simulink model "PID_controller"  (R2020a)
settings: Solver=VariableStepAuto  StartTime=0.0  StopTime=20  MaxStep=1e-3  RelTol=1e-3  EnableMultiTasking=on
settings Model: SILPILModeSetting=veronly  ExtModeTrigDuration=2  Creator=Administrator  LastModifiedBy=Administrator
settings OptimizationCC: BlockReduction=off  EnhancedBackFolding=on  PassReuseOutputArgsAs=Individual arguments  ZeroExternalMemoryAtStartup=off  ZeroInternalMemoryAtStartup=off  MaxStackSize=64  OptimizeBlockOrder=speed  DifferentSizesBufferReuse=on  OptimizationCustomize=off  EfficientTunableParamExpr=on
settings DebuggingCC: ParameterTunabilityLossMsg=error
settings HardwareCC: ProdBitPerInt=16  ProdBitPerPointer=16  ProdBitPerSizeT=16  ProdBitPerPtrDiffT=16  ProdLargestAtomicFloat=None  ProdWordSize=8  ProdHWDeviceType=Atmel->AVR
settings SFSimCC: MATLABDynamicMemAlloc=off
settings RTWCC: SystemTargetFile=ert.tlc  HardwareBoard=Arduino Uno  TLCOptions=-aInlineSetEventsForThisBaseRateFcn=TLC_FALSE -aSuppressMultiTaskScheduler=TLC_FALSE -aRateBasedStepFcn=1  TemplateMakefile=ert_default_tmf  Toolchain=Arduino AVR  BuildConfiguration=Faster Runs
settings CodeAppCC: ForceParamTrailComments=on  IgnoreCustomStorageClasses=off  OperatorAnnotations=on  SimulinkDataObjDesc=on  SFDataObjDesc=on  InsertBlockDesc=on
settings ERTTargetCC: SupportContinuousTime=on  SupportVariableSizeSignals=on  ExtModeStaticAllocSize=250

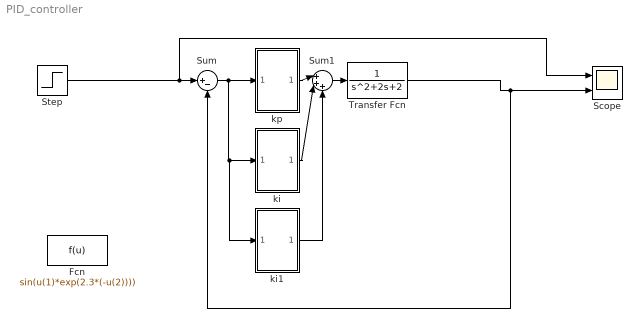
== system PID_controller ==
  Fcn : Fcn  Expr=sin(u(1)*exp(2.3*(-u(2))))
  Scope : Scope  NumInputPorts=2
  Step : Step  SampleTime=1
  Sum : Sum  Inputs=|+-
  Sum1 : Sum  Inputs=|+++
  Transfer Fcn : TransferFcn  Denominator=[1 2 2]
  ki : Subsystem
  ki1 : Subsystem
  kp : Subsystem
  wires:
  Step/1 -> Scope/1, Sum/1
  Transfer Fcn/1 -> Sum/2, Scope/2
  Sum/1 -> ki1/1(In1), ki/1(In1), kp/1(In1)
  kp/1(Out1) -> Sum1/1
  Sum1/1 -> Transfer Fcn/1
  ki/1(Out1) -> Sum1/2
  ki1/1(Out1) -> Sum1/3

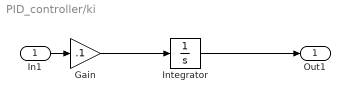
== system PID_controller/ki ==
  In1 : Inport
  Gain : Gain  Gain=.1
  Integrator : Integrator  InitialCondition=1
  Out1 : Outport
  wires:
  Gain/1 -> Integrator/1
  In1/1 -> Gain/1
  Integrator/1 -> Out1/1

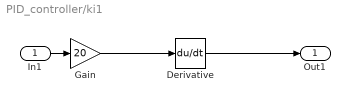
== system PID_controller/ki1 ==
  In1 : Inport
  Derivative : Derivative
  Gain : Gain  Gain=20
  Out1 : Outport
  wires:
  Derivative/1 -> Out1/1
  In1/1 -> Gain/1
  Gain/1 -> Derivative/1

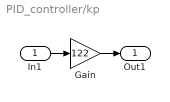
== system PID_controller/kp ==
  In1 : Inport
  Gain : Gain  Gain=122
  Out1 : Outport
  wires:
  In1/1 -> Gain/1
  Gain/1 -> Out1/1
